simulink model "ParkClarke_transform"  (R2023b)
settings: Solver=VariableStepAuto  StartTime=0.0  StopTime=0.1  MaxStep=0.0001  RelTol=1e-3
libraries: mcbcontrolslib x1, spspowerguiLib x1
settings Model: Creator=Son  LastModifiedBy=Son

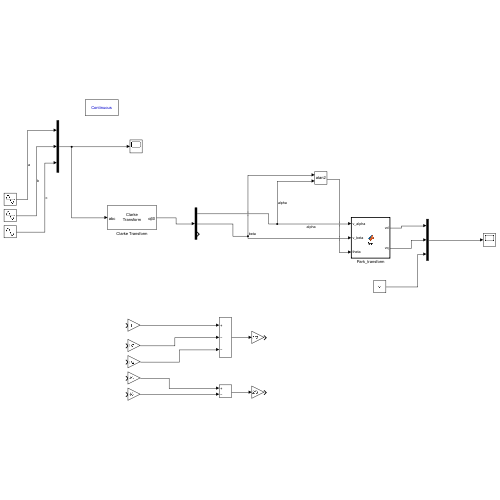
[thumbnail: Simulink's stored preview of the top-level diagram]
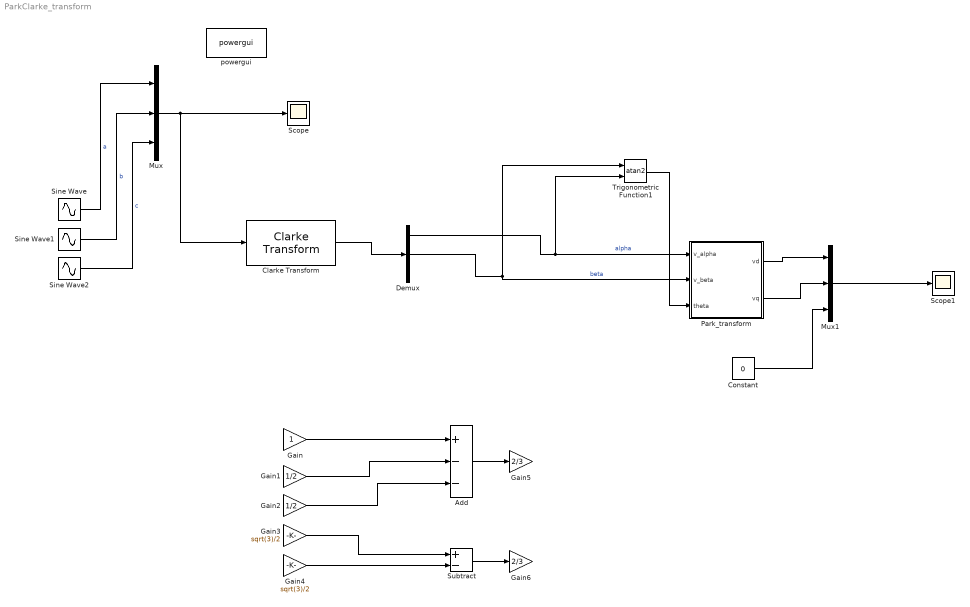
== system ParkClarke_transform ==
  Add : Sum  Inputs=+--
  Clarke Transform : mcbcontrolslib/Clarke Transform  VariantControl=Variant2  PhaseInput=Three inputs  EnPowerInv=off
      settings: LibrarySourceBlock=mcbhdllib/Controls/Math Transforms/Clarke Transform
  Constant : Constant  Value=0
  Demux : Demux  Outputs=3
  Gain : Gain
  Gain1 : Gain  Gain=1/2
  Gain2 : Gain  Gain=1/2
  Gain3 : Gain  Gain=sqrt(3)/2
  Gain4 : Gain  Gain=sqrt(3)/2
  Gain5 : Gain  Gain=2/3
  Gain6 : Gain  Gain=2/3
  Mux : Mux  Inputs=3
  Mux1 : Mux  Inputs=3
  Park_transform : MATLAB Function  TreatAsAtomicUnit=on
  Scope : Scope
  Scope1 : Scope
  Sine Wave : Sin  Frequency=2*pi*50  SampleTime=0
  Sine Wave1 : Sin  Frequency=2*pi*50  Phase=(2*pi)/3  SampleTime=0
  Sine Wave2 : Sin  Frequency=2*pi*50  Phase=-2*pi/3  SampleTime=0
  Subtract : Sum  Inputs=+-
  Trigonometric Function1 : Trigonometry  Operator=atan2
  powergui : spspowerguiLib/powergui  Priority=1  SimulationMode=Continuous  SampleTime=1e-4  frequency=60  Iterations=50  frequencyindice=60  Pbase=100e6  ErrMax=1e-4  UnitsV=kV  UnitsW=MW  buscounter=0  FunctionMessages=off  echomessages=off  EnableUseOfTLC=off  CurrentSourceSwitches=off  DisableSnubberDevices=off  DisableRonSwitches=off  DisableVfSwitches=off  DisplayEquations=off  AutomaticDiscreteSolvers=off  SolverType=Tustin/Backward Euler (TBE)  Interpol=off  ExternalGateDelay=off  methode=off  Ts=100  x0status=blocks  SPID=on  SwTol=0  HookPort=off  NonlinearTolerance=1e-4  nMaxIteration=100  ContinueOnMaxIteration=off  RestoreLinks=warning  ResistiveCurrentMeasurement=off  Frange=[0:2:500]  Ylog=off  Xlog=on  ShowGrid=off  save=off  variable=ZData  structure=0  ZoomFFT=off  StartTime=0.0  cycles=1  DisplayStyle=1  fundamental=60  FreqAxis=off  MaxFrequency=1000  frequencyindicesteady=1  RmsSteady=1  display=off
  wires:
  Sine Wave1/1 -> Mux/2  "b"
  Sine Wave2/1 -> Mux/3  "c"
  Sine Wave/1 -> Mux/1  "a"
  Mux/1 -> Clarke Transform/1, Scope/1
  Gain/1 -> Add/1
  Gain1/1 -> Add/2
  Gain2/1 -> Add/3
  Gain3/1 -> Subtract/1
  Gain4/1 -> Subtract/2
  Add/1 -> Gain5/1
  Subtract/1 -> Gain6/1
  Trigonometric Function1/1 -> Park_transform/3(theta)
  Park_transform/1(vd) -> Mux1/1
  Park_transform/2(vq) -> Mux1/2
  Constant/1 -> Mux1/3
  Clarke Transform/1 -> Demux/1
  Demux/1 -> Trigonometric Function1/2, Park_transform/1(v_alpha)  "alpha"
  Demux/2 -> Trigonometric Function1/1, Park_transform/2(v_beta)  "beta"
  Mux1/1 -> Scope1/1

== matlab function ParkClarke_transform/Park_transform ==
  data: v_alpha input; v_beta input; theta input; vd output; vq output
function [vd, vq] =  fcn(v_alpha, v_beta, theta)

vd = cos(theta) * v_alpha + sin(theta) * v_beta;
vq = -sin(theta) * v_alpha + cos(theta) * v_beta;
